simulink model "c2_6_2jiangweiguancekongzhiqi"  (R2019b)
settings: Solver=VariableStepAuto  StartTime=0.0  StopTime=30  RelTol=1e-3
settings Model: Creator=wy151  LastModifiedBy=wy151

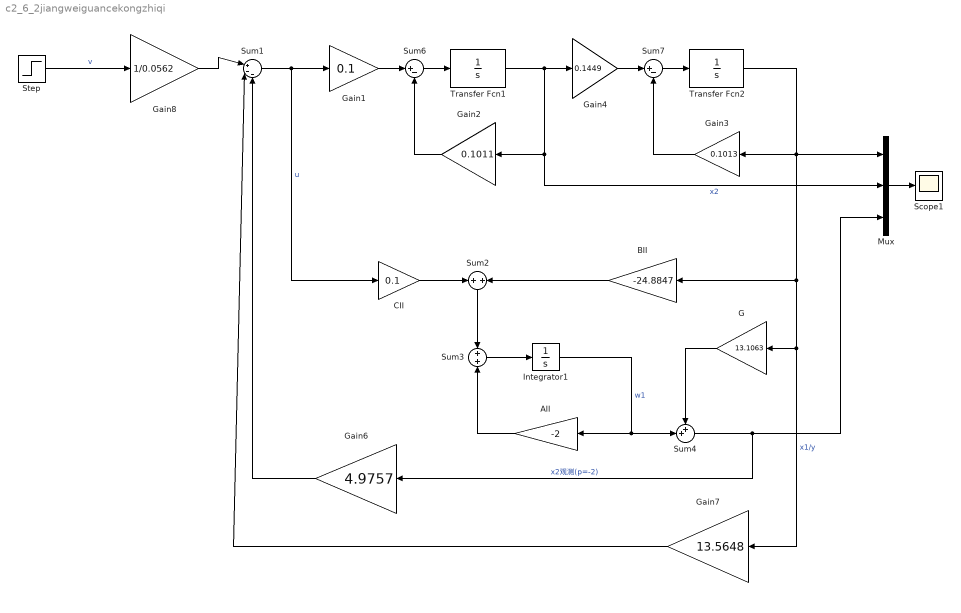
== system c2_6_2jiangweiguancekongzhiqi ==
  AII : Gain  Gain=-2
  BII : Gain  Gain=-24.8847
  CII : Gain  Gain=0.1
  G : Gain  Gain=13.1063
  Gain1 : Gain  Gain=0.1
  Gain2 : Gain  Gain=0.1011
  Gain3 : Gain  Gain=0.1013
  Gain4 : Gain  Gain=0.1449
  Gain6 : Gain  Gain=4.9757
  Gain7 : Gain  Gain=13.5648
  Gain8 : Gain  Gain=1/0.0562
  Integrator1 : Integrator
  Mux : Mux  Inputs=3
  Scope1 : Scope
  Step : Step  SampleTime=0
  Sum1 : Sum  Inputs=|+--
  Sum2 : Sum  Inputs=+|+
  Sum3 : Sum  Inputs=+|+
  Sum4 : Sum  Inputs=++|
  Sum6 : Sum  Inputs=|+-
  Sum7 : Sum  Inputs=|+-
  Transfer Fcn1 : TransferFcn  Denominator=[1 0]
  Transfer Fcn2 : TransferFcn  Denominator=[1 0]
  wires:
  Step/1 -> Gain8/1  "v"
  Gain7/1 -> Sum1/2
  Gain6/1 -> Sum1/3
  AII/1 -> Sum3/2
  Integrator1/1 -> Sum4/2, AII/1  "w1"
  Gain4/1 -> Sum7/1
  Sum6/1 -> Transfer Fcn1/1
  Sum2/1 -> Sum3/1
  Sum7/1 -> Transfer Fcn2/1
  BII/1 -> Sum2/2
  Sum4/1 -> Gain6/1, Mux/3  "x2观测(p=-2)"
  G/1 -> Sum4/1
  Gain3/1 -> Sum7/2
  Gain1/1 -> Sum6/1
  Transfer Fcn1/1 -> Mux/2, Gain2/1, Gain4/1  "x2"
  Gain2/1 -> Sum6/2
  Transfer Fcn2/1 -> Mux/1, Gain7/1, G/1, BII/1, Gain3/1  "x1/y"
  CII/1 -> Sum2/1
  Sum3/1 -> Integrator1/1
  Sum1/1 -> CII/1, Gain1/1  "u"
  Mux/1 -> Scope1/1
  Gain8/1 -> Sum1/1
